simulink model "Case4"  (R2023b)
settings: Solver=VariableStepAuto  StartTime=0.0  StopTime=10.0  RelTol=1e-3
settings Model: Creator=DarianMuresan  LastModifiedBy=DarianMuresan

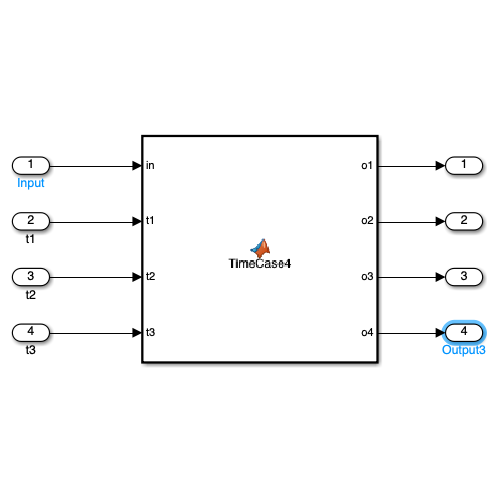
[thumbnail: Simulink's stored preview of the top-level diagram]
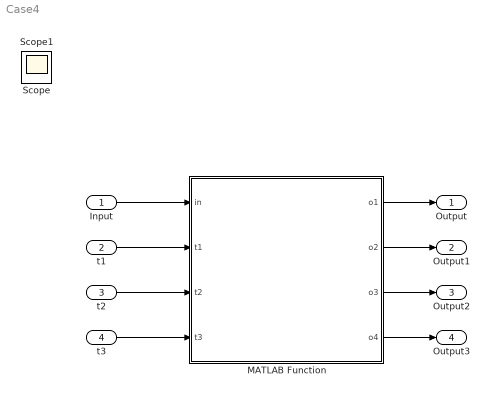
== system Case4 ==
  Input : Inport
  t1 : Inport  Port=2
  t2 : Inport  Port=3
  t3 : Inport  Port=4
  MATLAB Function : MATLAB Function  TreatAsAtomicUnit=on
  Output : Outport
  Output1 : Outport  Port=2
  Output2 : Outport  Port=3
  Output3 : Outport  Port=4
  Scope : Scope
  Scope1 : Scope
  wires:
  MATLAB Function/1(o1) -> Output/1
  MATLAB Function/2(o2) -> Output1/1
  MATLAB Function/3(o3) -> Output2/1
  MATLAB Function/4(o4) -> Output3/1
  Input/1 -> MATLAB Function/1(in)
  t1/1 -> MATLAB Function/2(t1)
  t2/1 -> MATLAB Function/3(t2)
  t3/1 -> MATLAB Function/4(t3)

== matlab function Case4/MATLAB Function ==
  data: in input; o1 output; t1 input; o2 output; o3 output; o4 output; t2 input; t3 input
function [o1,o2,o3,o4] = TimeCase4(in,t1,t2,t3)

% Method to demux input into one of 4 possible outputs based on
% probabilities.
%
% t1, t2, t3 are threshold bounds between 0 and 100
% that are used as follows:
% x = rand*100;
% 0  <= x < t1  => o1
% t1 <= x < t2  => o2
% t2 <= x < t3  => o3
% t3 <= x <=100 => o4
% 
% A non-valid output is negative
%
% Written by: Darian Muresan
% Last Modified: 10/17/2023

o1 = -1;
o2 = -1;
o3 = -1;
o4 = -1;

%rng('shuffle');
x = rand*100;

if 0  <= x && x < t1
    o1 = in;
elseif t1 <= x && x < t2
    o2 = in;
elseif t2 <= x && x < t3
    o3 = in;
else
    o4 = in;
end
